simulink model "bluetooth-controlled-sumo-robot-simulink"  (R2025b)
settings: Solver=VariableStepAuto  StartTime=0.0  StopTime=10.0  RelTol=1e-3
settings Model: Creator=20101  LastModifiedBy=20101

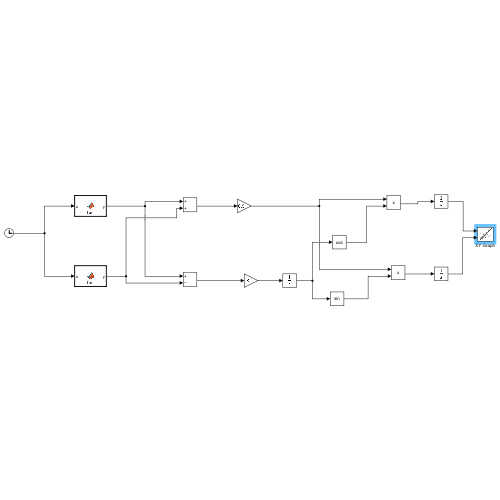
[thumbnail: Simulink's stored preview of the top-level diagram]
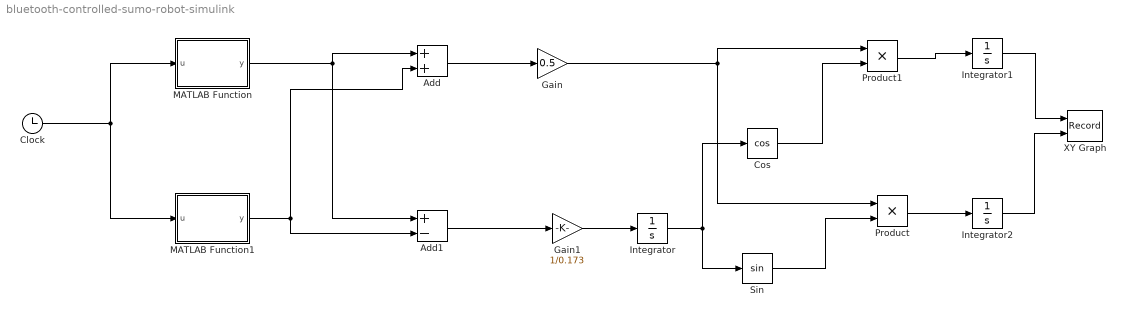
== system bluetooth-controlled-sumo-robot-simulink ==
  Add : Sum
  Add1 : Sum  Inputs=+-
  Clock : Clock
  Cos : Trigonometry  Operator=cos
  Gain : Gain  Gain=0.5
  Gain1 : Gain  Gain=1/0.173
  Integrator : Integrator
  Integrator1 : Integrator
  Integrator2 : Integrator
  MATLAB Function : MATLAB Function  TreatAsAtomicUnit=on
  MATLAB Function1 : MATLAB Function  TreatAsAtomicUnit=on
  Product : Product
  Product1 : Product
  Sin : Trigonometry
  XY Graph : Record  NumPorts=2.0  FileSettingsInternal="{\"entries\":[{\"content\":{\"excelSettings\":{\"content\":{},\"type\":\"Streamout.ExcelSettings\"},\"parquetSettings\":{\"content\":{},\"type\":\"Streamout.ParquetSettings\"}},\"type\":\"Streamout.FileSettingStorage\",\"uuid\":\"\"}],\"packageUris\":[\"http:\\/\\/schema.mathworks.com\\/mf0\\/streamout_blocks\\/R2020a\"],\"version\":\"1.0\"}"  FrameSettings=[0, 0]  Layout=[1 1]  SignalsInternal="{\"entries\":[{\"content\":{\"signals\":[{\"content\":{\"blockPath\":[],\"dimensions\":[1],\"domain\":\"\",\"lineColor\":\"#a2142f\",\"plots\":[ 1 ],\"port\":1,\"signalID\":1,\"signalName\":\"Integrator1\"},\"type\":\"RecordBlkView.Signal\",\"uuid\":\"\"},{\"content\":{\"blockPath\":[],\"dimensions\":[1],\"domain\":\"\",\"lineColor\":\"#139fff\",\"plots\":[ 1 ],\"port\":2,\"signalID\":2,\"signalName\":\"Integrator2\"},\"type\":\"RecordBlkView.Signal\",\"uuid\":\"\"}]},\"type\":\"RecordBlkView.InputSignals\",\"uuid\":\"\"}],\"packageUris\":[\"http:\\/\\/schema.mathworks.com\\/mf0\\/streamout_blocks\\/R2020a\"],\"version\":\"1.0\"}"  VisualizationBindings="{\"xyplotplugin\":{\"info\":[{\"series\":[{\"bindingParametersList\":[{\"parameter\":\"X-Axis\",\"signalID\":1,\"signalName\":\"Integrator1\"},{\"parameter\":\"Y-Axis\",\"signalID\":2,\"signalName\":\"Integrator2\"}],\"seriesID\":0}],\"subplotID\":1}]}}"  CompatibilityTag=XY
  wires:
  Clock/1 -> MATLAB Function1/1(u), MATLAB Function/1(u)
  MATLAB Function/1(y) -> Add1/1, Add/1
  MATLAB Function1/1(y) -> Add/2, Add1/2
  Add/1 -> Gain/1
  Add1/1 -> Gain1/1
  Gain1/1 -> Integrator/1
  Integrator/1 -> Sin/1, Cos/1
  Gain/1 -> Product/1, Product1/1
  Cos/1 -> Product1/2
  Sin/1 -> Product/2
  Product1/1 -> Integrator1/1
  Product/1 -> Integrator2/1
  Integrator1/1 -> XY Graph/1
  Integrator2/1 -> XY Graph/2

== matlab function bluetooth-controlled-sumo-robot-simulink/MATLAB Function ==
  data: u input; y output
function y = fcn(u)

if(u<=1)
    y=1.5;
elseif(u>1 && u<3)
    y=1.135;
elseif(u>3 && u<4)
    y=0.5;
else
    y=0;
end
end

== matlab function bluetooth-controlled-sumo-robot-simulink/MATLAB Function1 ==
  data: u input; y output
function y = fcn(u)

if(u<=1)
    y=1.5;
elseif(u>1 && u<3)
    y=0.864;
elseif(u>3 && u<4)
    y=0.5;
else
    y=0;
end
end
